simulink model "motorcycleHW"  (R2019a)
settings: Solver=FixedStepAuto  StartTime=0.0  StopTime=inf  RelTol=1e-3  EnableMultiTasking=on
PreLoadFcn:
  | createSensorBus;
  | Ts = 0.01;
  | Ts_wifi = 0.1;
libraries: mkrmotorcarrierlib x5, arduinosensorlib x1, simulink x1
settings Model: SimulationMode=external  ExtModeTrigDuration=2  Creator=bnewman  LastModifiedBy=mgovinda
settings DataIOCC: ReturnWorkspaceOutputs=off
settings OptimizationCC: PassReuseOutputArgsThreshold=0  MaxStackSize=64
settings DebuggingCC: ParameterTunabilityLossMsg=error  PregeneratedLibrarySubsystemCodeDiagnostic=none  ArithmeticOperatorsInVariantConditions=warning
settings HardwareCC: ProdBitPerPointer=32  ProdBitPerSizeT=32  ProdBitPerPtrDiffT=32  ProdLargestAtomicInteger=Long  ProdLargestAtomicFloat=Double  ProdWordSize=32  ProdHWDeviceType=ARM Compatible->ARM Cortex
settings SFSimCC: SimUseLocalCustomCode=off  MATLABDynamicMemAlloc=off
settings RTWCC: SystemTargetFile=ert.tlc  HardwareBoard=Arduino MKR WiFi 1010  TLCOptions=-aInlineSetEventsForThisBaseRateFcn=TLC_FALSE -aSuppressMultiTaskScheduler=TLC_FALSE -aRateBasedStepFcn=1  TemplateMakefile=ert_default_tmf  GenerateReport=on  RTWUseLocalCustomCode=off  Toolchain=Arduino ARM  BuildConfiguration=Faster Runs  LaunchReport=on
settings CodeAppCC: ForceParamTrailComments=on  OperatorAnnotations=on  MangleLength=10
settings ERTTargetCC: ERTCustomFileBanners=off  SupportContinuousTime=on  SupportNonInlinedSFcns=on  RemoveResetFunc=off  SupportVariableSizeSignals=on  ModelStepFunctionPrototypeControlCompliant=off  ExtModeStaticAllocSize=8192

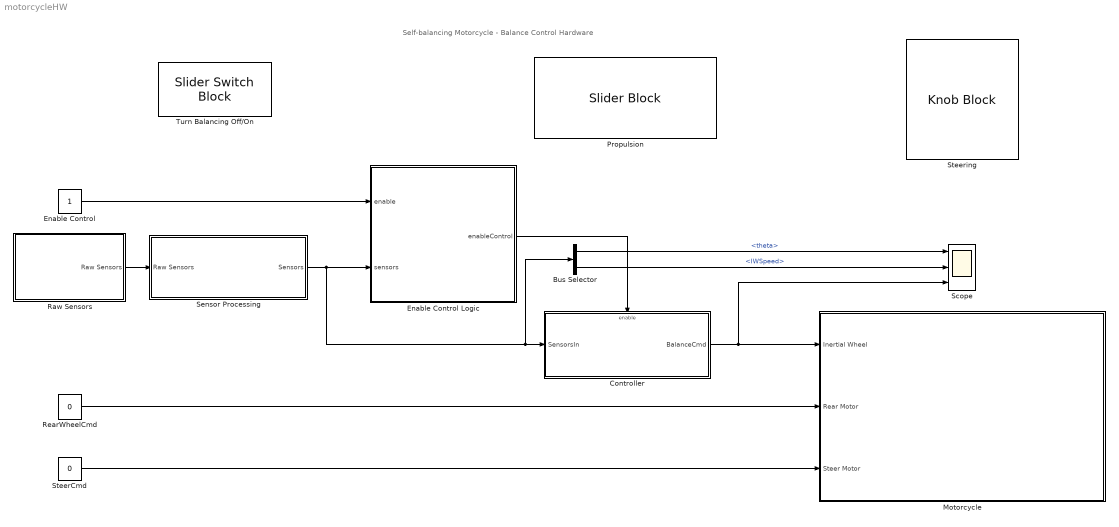
== system motorcycleHW ==
  note: Self-balancing Motorcycle - Balance Control Hardware
  Bus Selector : BusSelector  OutputSignals=theta,IWSpeed
  Controller : Subsystem
  Enable Control : Constant  SampleTime=Ts
  Enable Control Logic : Stateflow chart  TreatAsAtomicUnit=on
  Motorcycle : Subsystem
      mask Display: image('bikeHW.png');
  Propulsion : SliderBlock  LabelPosition=Hide  ScaleMin=-1  ScaleMax=1
  Raw Sensors : Subsystem
  RearWheelCmd : Constant  Value=0  SampleTime=Ts
  Scope : Scope  NumInputPorts=3
  Sensor Processing : Subsystem
  SteerCmd : Constant  Value=0  SampleTime=Ts
  Steering : KnobBlock  LabelPosition=Hide  ScaleMin=-30  ScaleMax=30
  Turn Balancing Off/On : SliderSwitchBlock  LabelPosition=Hide
      settings: Values={{'Off', 'On'}, [0 1]}
  wires:
  Enable Control/1 -> Enable Control Logic/1(enable)
  Controller/1(BalanceCmd) -> Scope/3, Motorcycle/1(Inertial Wheel)
  Enable Control Logic/1(enableControl) -> Controller/Enable
  Sensor Processing/1(Sensors) -> Enable Control Logic/2(sensors), Bus Selector/1, Controller/1(SensorsIn)
  Raw Sensors/1(Raw Sensors) -> Sensor Processing/1(Raw Sensors)
  RearWheelCmd/1 -> Motorcycle/2(Rear Motor)
  Bus Selector/1 -> Scope/1  "<theta>"
  Bus Selector/2 -> Scope/2  "<IWSpeed>"
  SteerCmd/1 -> Motorcycle/3(Steer Motor)

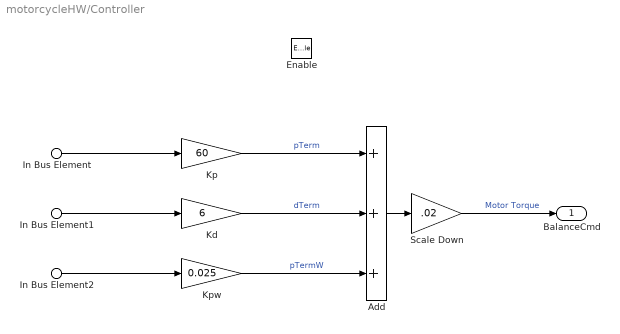
== system motorcycleHW/Controller ==
  In Bus Element : Inport  PortName=SensorsIn  Element=theta
  In Bus Element1 : Inport  PortName=SensorsIn  Element=thetaDot
  In Bus Element2 : Inport  PortName=SensorsIn  Element=IWSpeed
  Enable : EnablePort  StatesWhenEnabling=reset
  Add : Sum  Inputs=3
  Kd : Gain  Gain=6
  Kp : Gain  Gain=60
  Kpw : Gain  Gain=0.025
  Scale Down : Gain  Gain=.02
  BalanceCmd : Outport  OutputWhenDisabled=reset  InitialOutput=0
  wires:
  In Bus Element2/1 -> Kpw/1
  Scale Down/1 -> BalanceCmd/1  "Motor Torque"
  In Bus Element/1 -> Kp/1
  In Bus Element1/1 -> Kd/1
  Add/1 -> Scale Down/1
  Kd/1 -> Add/2  "dTerm"
  Kpw/1 -> Add/3  "pTermW"
  Kp/1 -> Add/1  "pTerm"

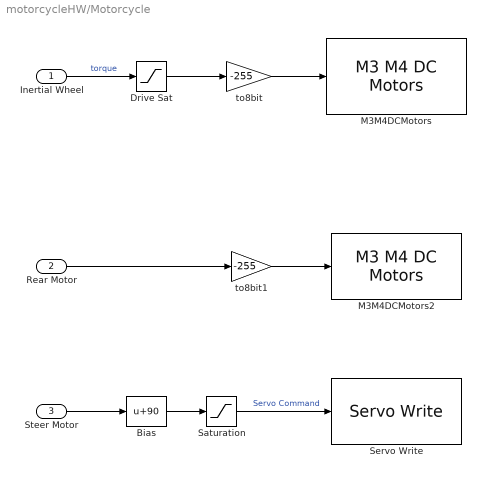
== system motorcycleHW/Motorcycle ==
  Inertial Wheel : Inport
  Rear Motor : Inport  Port=2
  Steer Motor : Inport  Port=3
  Bias : Bias  Bias=90
  Drive Sat : Saturate  UpperLimit=1  LowerLimit=-1
  M3M4DCMotors : mkrmotorcarrierlib/M3 M4 DC Motors  MotorNumber=M3
      settings: SourceProductName=Simulink Support for Arduino MKR Motor Shield
  M3M4DCMotors2 : mkrmotorcarrierlib/M3 M4 DC Motors  MotorNumber=M4
      settings: SourceProductName=Simulink Support for Arduino MKR Motor Carrier
  Saturation : Saturate  UpperLimit=120  LowerLimit=60
  Servo Write : mkrmotorcarrierlib/Servo Write  SlaveAddress=uint8( hex2dec( '66' ) )  blockPlatform=ARDUINO  MotorNumber=3  MotorCarrierPWMFreq=100
      settings: SourceProductName=Simulink Support for Arduino MKR Motor Shield
  to8bit : Gain  Gain=-255
  to8bit1 : Gain  Gain=-255
  wires:
  to8bit/1 -> M3M4DCMotors/1
  Drive Sat/1 -> to8bit/1
  Inertial Wheel/1 -> Drive Sat/1  "torque"
  Rear Motor/1 -> to8bit1/1
  to8bit1/1 -> M3M4DCMotors2/1
  Saturation/1 -> Servo Write/1  "Servo Command"
  Bias/1 -> Saturation/1
  Steer Motor/1 -> Bias/1

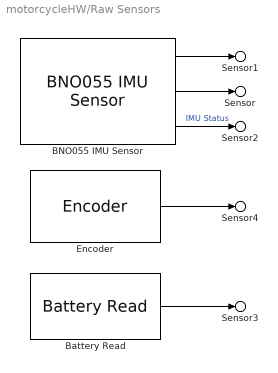
== system motorcycleHW/Raw Sensors ==
  BNO055 IMU Sensor : arduinosensorlib/BNO055 IMU Sensor  SlaveAddress=0x28  OperationMode=Fusion  Accel=off  AngularRate=on  MagField=off  EulerAngles=on  Quat=off  LinearAccel=off  GravityVector=off  AccelRange=4G  AccelBW=62.5 Hz  GyroRange=2000 dps  GyroBW=32 Hz  MagODR=10 Hz  SampleTime=0.01  blockPlatform=ARDUINO
      settings: SourceProductName=Simulink Support for Arduino Sensors
  Battery Read : mkrmotorcarrierlib/Battery Read  SlaveAddress=uint8( hex2dec( '66' ) )  blockPlatform=ARDUINO  SampleTime=0.01
      settings: SourceProductName=Simulink Support for Arduino MKR Motor Shield
  Encoder : mkrmotorcarrierlib/Encoder  SlaveAddress=uint8( hex2dec( '66' ) )  blockPlatform=ARDUINO  Encoder=1  ShowSpeed=off  ResetOption=on  SampleTime=Ts
      settings: SourceProductName=Simulink Support for Arduino MKR Motor Carrier
  Sensor : Outport  PortName=Raw Sensors  Element=Theta
  Sensor1 : Outport  PortName=Raw Sensors  Element=ThetaDot
  Sensor2 : Outport  PortName=Raw Sensors  Element=IMU_Status
  Sensor3 : Outport  PortName=Raw Sensors  Element=Battery
  Sensor4 : Outport  PortName=Raw Sensors  Element=EncCounts
  wires:
  Battery Read/1 -> Sensor3/1
  BNO055 IMU Sensor/1 -> Sensor1/1
  BNO055 IMU Sensor/3 -> Sensor2/1  "IMU Status"
  BNO055 IMU Sensor/2 -> Sensor/1
  Encoder/1 -> Sensor4/1

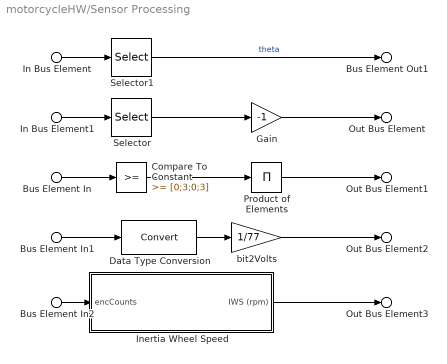
== system motorcycleHW/Sensor Processing ==
  Bus Element In : Inport  PortName=Raw Sensors  Element=IMU_Status
  In Bus Element : Inport  PortName=Raw Sensors  Element=Theta
  In Bus Element1 : Inport  PortName=Raw Sensors  Element=ThetaDot
  Bus Element In1 : Inport  PortName=Raw Sensors  Element=Battery
  Bus Element In2 : Inport  PortName=Raw Sensors  Element=EncCounts
  Compare To Constant : simulink/Logic and Bit Operations/Compare To Constant  relop=>=  const=[0;3;0;3]  OutDataTypeStr=boolean
  Data Type Conversion : DataTypeConversion
  Gain : Gain  Gain=-1
  Inertia Wheel Speed : Subsystem
  Product of Elements : Product  Inputs=*
  Selector : Selector  InputPortWidth=3  IndexOptions=Index vector (dialog)  Indices=2  OutputSizes=1
  Selector1 : Selector  InputPortWidth=3  IndexOptions=Index vector (dialog)  Indices=2  OutputSizes=1
  bit2Volts : Gain  Gain=1/77
  Bus Element Out1 : Outport  PortName=Sensors  Element=theta
  Out Bus Element : Outport  PortName=Sensors  Element=thetaDot
  Out Bus Element1 : Outport  PortName=Sensors  Element=imuCalibrated
  Out Bus Element2 : Outport  PortName=Sensors  Element=Volt
  Out Bus Element3 : Outport  PortName=Sensors  Element=IWSpeed
  wires:
  Selector/1 -> Gain/1
  In Bus Element1/1 -> Selector/1
  In Bus Element/1 -> Selector1/1
  Selector1/1 -> Bus Element Out1/1  "theta"
  Compare To Constant/1 -> Product of Elements/1
  Bus Element In/1 -> Compare To Constant/1
  Data Type Conversion/1 -> bit2Volts/1
  Bus Element In1/1 -> Data Type Conversion/1
  Bus Element In2/1 -> Inertia Wheel Speed/1(encCounts)
  Product of Elements/1 -> Out Bus Element1/1
  Gain/1 -> Out Bus Element/1
  Inertia Wheel Speed/1(IWS (rpm)) -> Out Bus Element3/1
  bit2Volts/1 -> Out Bus Element2/1

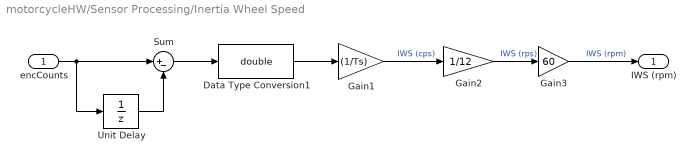
== system motorcycleHW/Sensor Processing/Inertia Wheel Speed ==
  encCounts : Inport
  Data Type Conversion1 : DataTypeConversion  OutDataTypeStr=double
  Gain1 : Gain  Gain=(1/Ts)
  Gain2 : Gain  Gain=1/12  OutDataTypeStr=double
  Gain3 : Gain  Gain=60  OutDataTypeStr=double
  Sum : Sum  Inputs=|+-
  Unit Delay : UnitDelay  SampleTime=-1  HasFrameUpgradeWarning=on
  IWS (rpm) : Outport
  wires:
  Gain2/1 -> Gain3/1  "IWS (rps)"
  Gain1/1 -> Gain2/1  "IWS (cps)"
  Gain3/1 -> IWS (rpm)/1  "IWS (rpm)"
  Unit Delay/1 -> Sum/2
  encCounts/1 -> Unit Delay/1, Sum/1
  Data Type Conversion1/1 -> Gain1/1
  Sum/1 -> Data Type Conversion1/1

== stateflow chart motorcycleHW/Enable Control Logic ==
  state checkIMUCalib [parallel]
    settings: executionOrder=1
    state imuNotCalibrated
      entry:
      isIMUCalibrated = false;
    state imuCalibrated
      entry:
      isIMUCalibrated = true;
    (default) -> imuNotCalibrated
    imuNotCalibrated -> imuCalibrated : [sensors.imuCalibrated == true]
  state checkFallen [parallel]
    du: t = sensors.theta;
    settings: executionOrder=3
    state Standing
      entry:
      isFallen = false;
    state Fallen
      entry:
      isFallen = true;
    (default) -> Standing
    Standing -> Fallen : [abs(t) >6]
    Fallen -> Standing : [abs(t) <6]
  state Running [parallel]
    settings: executionOrder=4
    state Waiting
      entry: enableControl = false
    state Running
      state On
        enableControl = true;
      state Off
        enableControl = false;
      Running.Running -> (junction 53) [order 1]
      (default) -> (junction 53)
      (junction 53) -> (junction 57) [order 1] : [isIMUCalibrated && (isBatteryOK) && not(isFallen)]
      (junction 53) -> Off [order 2]
      (junction 57) -> On
    (default) -> Waiting
    Waiting -> Running.Running : [enable]
    Running.Running -> Waiting [order 1] : [not(enable)]
  state checkBattery [parallel]
    settings: executionOrder=2
    state batteryNotCharged
      entry:
      isBatteryOK = false;
    state batteryCharged
      entry:
      isBatteryOK = true;
    (default) -> batteryNotCharged
    batteryCharged -> batteryNotCharged : [sensors.Volt < 11]
    batteryNotCharged -> batteryCharged : [sensors.Volt >= 11]
  data: enable input; sensors input Bus: sensorBus size=1; isBatteryOK local; enableControl output; isFallen local; isIMUCalibrated local; t local
